simulink model "SF007A_SysFricLrng"  (R2013b)
settings: Solver=FixedStepDiscrete  SolverMode=SingleTasking  StartTime=0.0  StopTime=1  FixedStep=0.002  RelTol=1e-3
PostLoadFcn:
  | , if any(exist('dsrtsu_mdlpostloadfcn', 'file') == [2, 3, 6]), try dsrtsu_mdlpostloadfcn('Execute', bdroot); catch fprintf('Error in PostLoadFcn (dsrtsu_mdlpostloadfcn) for model "%s":\n %s\n', bdroot, lasterr); end, end,
values from neighbouring files (symbols this model uses):
  ARCHGLBPRM_100MILLISEC_SEC_F32 = DataDict.Constant    [SF007A_SysFricLrng_DataDict.m]
  ARCHGLBPRM_10MILLISEC_SEC_F32 = DataDict.Constant    [SF007A_SysFricLrng_DataDict.m]
  ARCHGLBPRM_180OVERPI_ULS_F32 = DataDict.Constant    [SF007A_SysFricLrng_DataDict.m]
  CONV100MICROSECTOSEC_ULS_F32 = DataDict.Constant    [SF007A_SysFricLrng_DataDict.m]
  FLTINJ_SYSFRICLRNG_SYSFRICOFFS = DataDict.Constant    [SF007A_SysFricLrng_DataDict.m]
  FricLrngData = DataDict.NVM    [SF007A_SysFricLrng_DataDict.m]
  HWPTNUM_CNT_U08 = DataDict.Constant    [SF007A_SysFricLrng_DataDict.m]
  HWPTNUMSUB1_CNT_U08 = DataDict.Constant    [SF007A_SysFricLrng_DataDict.m]
  HWVELDECDIR_ULS_U08 = DataDict.Constant    [SF007A_SysFricLrng_DataDict.m]
  HWVELINCDIR_ULS_U08 = DataDict.Constant    [SF007A_SysFricLrng_DataDict.m]
  IDXCALCNSCAGFAC_ULS_U08 = DataDict.Constant    [SF007A_SysFricLrng_DataDict.m]
  IDXSELN1_ULS_U08 = DataDict.Constant    [SF007A_SysFricLrng_DataDict.m]
  IDXSELN2_ULS_U08 = DataDict.Constant    [SF007A_SysFricLrng_DataDict.m]
  IDXSELN3_ULS_U08 = DataDict.Constant    [SF007A_SysFricLrng_DataDict.m]
  LRNGENASCAFAC_MILLISEC_U32 = DataDict.Constant    [SF007A_SysFricLrng_DataDict.m]
  SCAGFACQUARTER_CNT_F32 = DataDict.Constant    [SF007A_SysFricLrng_DataDict.m]
  SCAGFACTEN_CNT_U16 = DataDict.Constant    [SF007A_SysFricLrng_DataDict.m]
  SCAGFACVEHLATA_MTRPERSECSQD_F32 = DataDict.Constant    [SF007A_SysFricLrng_DataDict.m]
  SECIDXSELN_ULS_U08 = DataDict.Constant    [SF007A_SysFricLrng_DataDict.m]
  SysFricLrngBasLineEolFric = DataDict.Calibration    [SF007A_SysFricLrng_DataDict.m]
  SysFricLrngBasLineFric = DataDict.Calibration    [SF007A_SysFricLrng_DataDict.m]
  SysFricLrngBasLineHys = DataDict.Calibration    [SF007A_SysFricLrng_DataDict.m]
  SysFricLrngBasLineRngCntr = DataDict.Calibration    [SF007A_SysFricLrng_DataDict.m]
  SysFricLrngEolFricDifScagFac = DataDict.Calibration    [SF007A_SysFricLrng_DataDict.m]
  SysFricLrngFricChgWght = DataDict.Calibration    [SF007A_SysFricLrng_DataDict.m]
  SysFricLrngFricDiagcThd = DataDict.Calibration    [SF007A_SysFricLrng_DataDict.m]
  SysFricLrngFricDiagcTiThd = DataDict.Calibration    [SF007A_SysFricLrng_DataDict.m]
  SysFricLrngFricHysHwAgPt = DataDict.Calibration    [SF007A_SysFricLrng_DataDict.m]
  SysFricLrngGain = DataDict.Calibration    [SF007A_SysFricLrng_DataDict.m]
  SysFricLrngHwPosnAuthyThd = DataDict.Calibration    [SF007A_SysFricLrng_DataDict.m]
  SysFricLrngHwVelConstrLim = DataDict.Calibration    [SF007A_SysFricLrng_DataDict.m]
  SysFricLrngHwVelHiLim = DataDict.Calibration    [SF007A_SysFricLrng_DataDict.m]
  SysFricLrngHwVelLoLim = DataDict.Calibration    [SF007A_SysFricLrng_DataDict.m]
  SysFricLrngIgnCycFricChgLim = DataDict.Calibration    [SF007A_SysFricLrng_DataDict.m]
  SysFricLrngLatAHiLim = DataDict.Calibration    [SF007A_SysFricLrng_DataDict.m]
  SysFricLrngLatALoLim = DataDict.Calibration    [SF007A_SysFricLrng_DataDict.m]
  SysFricLrngMaskVehSpd = DataDict.Calibration    [SF007A_SysFricLrng_DataDict.m]
  SysFricLrngRngCntrThd = DataDict.Calibration    [SF007A_SysFricLrng_DataDict.m]
  SysFricLrngThd = DataDict.Calibration    [SF007A_SysFricLrng_DataDict.m]
  SysFricLrngTHiLim = DataDict.Calibration    [SF007A_SysFricLrng_DataDict.m]
  SysFricLrngTLoLim = DataDict.Calibration    [SF007A_SysFricLrng_DataDict.m]
  SysFricLrngVehSpd = DataDict.Calibration    [SF007A_SysFricLrng_DataDict.m]
  SYSFRICOFFSLIM_HWNWTMTR_F32 = DataDict.Constant    [SF007A_SysFricLrng_DataDict.m]
  VEHSPDPTNUM1_ULS_U08 = DataDict.Constant    [SF007A_SysFricLrng_DataDict.m]
  VEHSPDPTNUM2_ULS_U08 = DataDict.Constant    [SF007A_SysFricLrng_DataDict.m]
undefined symbols (not defined in the file or in its folder): NtcNr1, NtcSts1, SysFricLrngOperMod1
libraries: Fil x19, simulink x17, NxtrLim x10, NxtrAbslt x3, NxtrNvM x2, FixdToFloat x2, FloatToFixd x1, LnrIntrpn x1
(part 7 of 7)

== system SF007A_SysFricLrng/SysFricLrng/SysFricLrngPer1/RunningAndCalibrationModes/FricLearning/Calculate Average Friction/Raw Average Calculation/Update LPF/InitAvrgFricLpFil3 ==
  RawAvgFric : Inport
  Action Port : ActionPort  ActionType=case
  CopyRight2 : Subsystem  Description=|  mask(Copyright Information){none=on}
      | Copyright info block.                                               
      |                                                                     
      | Place copyright information at the top of every subsystem in design.
      mask prompts: none "No parameters"
      mask help: Place copyright information at the top of every subsystem in design.
      mask Display:
      | NxtrConf = 'Nexteer Confidential';
      | 
      | sys = bdroot; %handle for the current model ("system")
      | first = get_param(sys,'Created');
      | first = first(end-3:end);  %year is last four digits
      | 
      | last = get_param(sys,'LastModifiedDate');
      | if isempty(last)
      |     last = datestr(now,'yyyy');
      | else
      |     last = last(end-3:end);
      | end
      | 
      | if strcmp(first,last)
      |     fprintf('%s -- Copyright %s Nexteer',NxtrConf,first)
      | else
      |     fprintf('%s -- %s%s- %s Nexteer',NxtrConf,char(169),first,last)
      | end
  FilLpUpdOutp : Subsystem  mask(FilLpUpdOutp){StVar=AvrgFricLpFil3}
      mask prompts: StVar "State Variable:"
      mask help: Simulink implementation of the LPF_OpUpdate_f32_m macro.
      mask init: same as SF007A_SysFricLrng/SysFricLrng/SysFricLrngPer1/RunningAndCalibrationModes/Running Mode/If Action Subsystem/BlendingFricChg/FilLpUpdOutp
      settings: AttributesFormatString=StVar: %<StVar>
      mask Display:
      | port_label('input',1,'Inp')
      | port_label('output',1,'Outp')
      | text(0.2,0.8,'FilLpUpdOutp')
  FiltAvgFric : Outport
  wires:
  RawAvgFric/1 -> FilLpUpdOutp/1(Input)
  FilLpUpdOutp/1(Out1) -> FiltAvgFric/1

== system SF007A_SysFricLrng/SysFricLrng/SysFricLrngPer1/RunningAndCalibrationModes/FricLearning/Calculate Average Friction/Raw Average Calculation/Update LPF/InitAvrgFricLpFil4 ==
  RawAvgFric : Inport
  Action Port : ActionPort  ActionType=default
  CopyRight2 : Subsystem  Description=|  mask(Copyright Information){none=on}
      | Copyright info block.                                               
      |                                                                     
      | Place copyright information at the top of every subsystem in design.
      mask prompts: none "No parameters"
      mask help: Place copyright information at the top of every subsystem in design.
      mask Display:
      | NxtrConf = 'Nexteer Confidential';
      | 
      | sys = bdroot; %handle for the current model ("system")
      | first = get_param(sys,'Created');
      | first = first(end-3:end);  %year is last four digits
      | 
      | last = get_param(sys,'LastModifiedDate');
      | if isempty(last)
      |     last = datestr(now,'yyyy');
      | else
      |     last = last(end-3:end);
      | end
      | 
      | if strcmp(first,last)
      |     fprintf('%s -- Copyright %s Nexteer',NxtrConf,first)
      | else
      |     fprintf('%s -- %s%s- %s Nexteer',NxtrConf,char(169),first,last)
      | end
  FilLpUpdOutp : Subsystem  mask(FilLpUpdOutp){StVar=AvrgFricLpFil4}
      mask prompts: StVar "State Variable:"
      mask help: Simulink implementation of the LPF_OpUpdate_f32_m macro.
      mask init: same as SF007A_SysFricLrng/SysFricLrng/SysFricLrngPer1/RunningAndCalibrationModes/Running Mode/If Action Subsystem/BlendingFricChg/FilLpUpdOutp
      settings: AttributesFormatString=StVar: %<StVar>
      mask Display:
      | port_label('input',1,'Inp')
      | port_label('output',1,'Outp')
      | text(0.2,0.8,'FilLpUpdOutp')
  FiltAvgFric : Outport
  wires:
  RawAvgFric/1 -> FilLpUpdOutp/1(Input)
  FilLpUpdOutp/1(Out1) -> FiltAvgFric/1

== system SF007A_SysFricLrng/SysFricLrng/SysFricLrngPer1/RunningAndCalibrationModes/FricLearning/Range Counter Manager/Range Counter Control1/UpdateBaselineFric/CopyRight2 ==

== system SF007A_SysFricLrng/SysFricLrng/SysFricLrngPer1/RunningAndCalibrationModes/FricLearning/Range Counter Manager/Range Counter Threshold Calculation/Do Nothig/CopyRight2 ==

== system SF007A_SysFricLrng/SysFricLrng/SysFricLrngPer1/RunningAndCalibrationModes/FricLearning/Range Counter Manager/Range Counter Threshold Calculation/RangeCounterThreshExceeded/CopyRight2 ==

== system SF007A_SysFricLrng/SysFricLrng/SysFricLrngPer1/RunningAndCalibrationModes/LearningConstraint/ColTqconstraint/ColTqAryCalcn/12 Delay's Execution/CopyRight2 ==

== system SF007A_SysFricLrng/SysFricLrng/SysFricLrngPer1/RunningAndCalibrationModes/LearningConstraint/HwAngConstraint/Handwheel Angle Buffer/12 Delay's Execution/CopyRight2 ==

== system SF007A_SysFricLrng/SysFricLrng/SysFricLrngPer1/RunningAndCalibrationModes/LearningConstraint/HwVelConstraint/Handwheel Velocity Buffer/12 Delay's Execution/CopyRight2 ==

== system SF007A_SysFricLrng/SysFricLrng/SysFricLrngPer1/RunningAndCalibrationModes/LearningConstraint/HwVelConstraint/Range_Monotonicity Calculation/ AllGTZ/CopyRight2 ==

== system SF007A_SysFricLrng/SysFricLrng/SysFricLrngPer1/RunningAndCalibrationModes/LearningConstraint/HwVelConstraint/Range_Monotonicity Calculation/AllLTZ/CopyRight2 ==

== system SF007A_SysFricLrng/SysFricLrng/SysFricLrngPer1/RunningAndCalibrationModes/FricLearning/Calculate Average Friction/NTC FAIL/GetTiSpan100MicroSec32bit/No wrapping/CopyRight2 ==

== system SF007A_SysFricLrng/SysFricLrng/SysFricLrngPer1/RunningAndCalibrationModes/FricLearning/Calculate Average Friction/NTC FAIL/GetTiSpan100MicroSec32bit/Wrapping/CopyRight2 ==

== system SF007A_SysFricLrng/SysFricLrng/SysFricLrngPer1/RunningAndCalibrationModes/FricLearning/Calculate Average Friction/NTC FAIL/NTCFAIL/SetNtcSts/SetNtcSts ==
  note: Note:
      |
      | - "ISO Fault Debounce Design" Simulink block intent to use here for Simulation purpose only. Do not Code this block
  NtcNr : Inport
  NtcStInfo : Inport  Port=2
  NtcSts : Inport  Port=3
  DebStep : Inport  Port=4
  CopyRight2 : Subsystem  Description=|  mask(Copyright Information){none=on}
      | Copyright info block.                                               
      |                                                                     
      | Place copyright information at the top of every subsystem in design.
      mask prompts: none "No parameters"
      mask help: Place copyright information at the top of every subsystem in design.
      mask Display:
      | NxtrConf = 'Nexteer Confidential';
      | 
      | sys = bdroot; %handle for the current model ("system")
      | first = get_param(sys,'Created');
      | first = first(end-3:end);  %year is last four digits
      | 
      | last = get_param(sys,'LastModifiedDate');
      | if isempty(last)
      |     last = datestr(now,'yyyy');
      | else
      |     last = last(end-3:end);
      | end
      | 
      | if strcmp(first,last)
      |     fprintf('%s -- Copyright %s Nexteer',NxtrConf,first)
      | else
      |     fprintf('%s -- %s%s- %s Nexteer',NxtrConf,char(169),first,last)
      | end
  Data Store Write : DataStoreWrite  DataStoreName=Ntc0X0A2Qlfr
  Data Type Conversion4 : DataTypeConversion  OutDataTypeStr=Enum: SigQlfr1
  Ground : Ground
  ISO Fault Debounce Design : Stateflow chart  TreatAsAtomicUnit=on
      settings: AttributesFormatString=|
      | Simulation Purpose Only.
      | Do Not Code this block
      | Diagnostic Manager Owns this requirement
  Terminator : Terminator
  Terminator1 : Terminator
  wires:
  NtcStInfo/1 -> Terminator1/1
  NtcNr/1 -> Terminator/1
  DebStep/1 -> ISO Fault Debounce Design/2(DebStep)
  ISO Fault Debounce Design/1(Qualifier) -> Data Type Conversion4/1
  Ground/1 -> ISO Fault Debounce Design/3(SvcClr)
  Data Type Conversion4/1 -> Data Store Write/1
  NtcSts/1 -> ISO Fault Debounce Design/1(NtcSts)

== system SF007A_SysFricLrng/SysFricLrng/SysFricLrngPer1/RunningAndCalibrationModes/FricLearning/Calculate Average Friction/NTC PASS /SetNtcSts/SetNtcSts/CopyRight2 ==

== system SF007A_SysFricLrng/SysFricLrng/SysFricLrngPer1/RunningAndCalibrationModes/FricLearning/Calculate Average Friction/Raw Average Calculation/Update LPF/InitAvrgFricLpFil1/CopyRight2 ==

== system SF007A_SysFricLrng/SysFricLrng/SysFricLrngPer1/RunningAndCalibrationModes/FricLearning/Calculate Average Friction/Raw Average Calculation/Update LPF/InitAvrgFricLpFil1/FilLpUpdOutp ==
  Input : Inport
  Add : Sum
  Data Store Read : DataStoreRead  DataStoreName=AvrgFricLpFil1  DataStoreElements=AvrgFricLpFil1.FilSt#AvrgFricLpFil1.FilGain
  Data Store Write : DataStoreWrite  DataStoreName=AvrgFricLpFil1  DataStoreElements=AvrgFricLpFil1.FilSt
  Display1 : Display
  Display2 : Display
  Product : Product
  Subtract : Sum  Inputs=+-
  Out1 : Outport  OutDataTypeStr=single
  wires:
  Data Store Read/2 -> Display1/1, Product/2
  Add/1 -> Out1/1, Data Store Write/1
  Product/1 -> Add/2
  Subtract/1 -> Product/1
  Input/1 -> Subtract/1
  Data Store Read/1 -> Display2/1, Subtract/2, Add/1

== system SF007A_SysFricLrng/SysFricLrng/SysFricLrngPer1/RunningAndCalibrationModes/FricLearning/Calculate Average Friction/Raw Average Calculation/Update LPF/InitAvrgFricLpFil2/CopyRight2 ==

== system SF007A_SysFricLrng/SysFricLrng/SysFricLrngPer1/RunningAndCalibrationModes/FricLearning/Calculate Average Friction/Raw Average Calculation/Update LPF/InitAvrgFricLpFil2/FilLpUpdOutp ==
  Input : Inport
  Add : Sum
  Data Store Read : DataStoreRead  DataStoreName=AvrgFricLpFil2  DataStoreElements=AvrgFricLpFil2.FilSt#AvrgFricLpFil2.FilGain
  Data Store Write : DataStoreWrite  DataStoreName=AvrgFricLpFil2  DataStoreElements=AvrgFricLpFil2.FilSt
  Display1 : Display
  Display2 : Display
  Product : Product
  Subtract : Sum  Inputs=+-
  Out1 : Outport  OutDataTypeStr=single
  wires:
  Data Store Read/2 -> Display1/1, Product/2
  Add/1 -> Out1/1, Data Store Write/1
  Product/1 -> Add/2
  Subtract/1 -> Product/1
  Input/1 -> Subtract/1
  Data Store Read/1 -> Display2/1, Subtract/2, Add/1

== system SF007A_SysFricLrng/SysFricLrng/SysFricLrngPer1/RunningAndCalibrationModes/FricLearning/Calculate Average Friction/Raw Average Calculation/Update LPF/InitAvrgFricLpFil3/CopyRight2 ==

== system SF007A_SysFricLrng/SysFricLrng/SysFricLrngPer1/RunningAndCalibrationModes/FricLearning/Calculate Average Friction/Raw Average Calculation/Update LPF/InitAvrgFricLpFil3/FilLpUpdOutp ==
  Input : Inport
  Add : Sum
  Data Store Read : DataStoreRead  DataStoreName=AvrgFricLpFil3  DataStoreElements=AvrgFricLpFil3.FilSt#AvrgFricLpFil3.FilGain
  Data Store Write : DataStoreWrite  DataStoreName=AvrgFricLpFil3  DataStoreElements=AvrgFricLpFil3.FilSt
  Display1 : Display
  Display2 : Display
  Product : Product
  Subtract : Sum  Inputs=+-
  Out1 : Outport  OutDataTypeStr=single
  wires:
  Data Store Read/2 -> Display1/1, Product/2
  Add/1 -> Out1/1, Data Store Write/1
  Product/1 -> Add/2
  Subtract/1 -> Product/1
  Input/1 -> Subtract/1
  Data Store Read/1 -> Display2/1, Subtract/2, Add/1

== system SF007A_SysFricLrng/SysFricLrng/SysFricLrngPer1/RunningAndCalibrationModes/FricLearning/Calculate Average Friction/Raw Average Calculation/Update LPF/InitAvrgFricLpFil4/CopyRight2 ==

== system SF007A_SysFricLrng/SysFricLrng/SysFricLrngPer1/RunningAndCalibrationModes/FricLearning/Calculate Average Friction/Raw Average Calculation/Update LPF/InitAvrgFricLpFil4/FilLpUpdOutp ==
  Input : Inport
  Add : Sum
  Data Store Read : DataStoreRead  DataStoreName=AvrgFricLpFil4  DataStoreElements=AvrgFricLpFil4.FilSt#AvrgFricLpFil4.FilGain
  Data Store Write : DataStoreWrite  DataStoreName=AvrgFricLpFil4  DataStoreElements=AvrgFricLpFil4.FilSt
  Display1 : Display
  Display2 : Display
  Product : Product
  Subtract : Sum  Inputs=+-
  Out1 : Outport  OutDataTypeStr=single
  wires:
  Data Store Read/2 -> Display1/1, Product/2
  Add/1 -> Out1/1, Data Store Write/1
  Product/1 -> Add/2
  Subtract/1 -> Product/1
  Input/1 -> Subtract/1
  Data Store Read/1 -> Display2/1, Subtract/2, Add/1

== system SF007A_SysFricLrng/SysFricLrng/SysFricLrngPer1/RunningAndCalibrationModes/FricLearning/Calculate Average Friction/NTC FAIL/NTCFAIL/SetNtcSts/SetNtcSts/CopyRight2 ==

== stateflow chart SF007A_SysFricLrng/SysFricLrng/SysFricLrngPer1/RunningAndCalibrationModes/FricLearning/Calculate Average Friction/NTC FAIL/NTCFAIL/SetNtcSts/SetNtcSts/ISO Fault Debounce Design ==
  note: NTCSTS_PASSD           (0)
      | NTCSTS_FAILD             (1)
      | NTCSTS_PREPASSD   (2)
      | NTCSTS_PREFAILD     (3)
      |
      | SIGQLFR_NORES        (0)
      | SIGQLFR_PASSD         (1)
      | SIGQLFR_FAILD           (2)
  note: Pass Loop
  note: Fail Loop
  note: 
  (default) -> (junction 89)
  (junction 89) -> (junction 95) [order 1] : [NtcSts ==3]
  (junction 89) -> (junction 93) [order 2] : [NtcSts ==2]
  (junction 89) -> (junction 141) [order 3] : [NtcSts ==1]
      | { ErrAcc = 32767;
      | Qualifier =2;
      |  }
  (junction 89) -> (junction 141) [order 4] : [NtcSts ==0]
      | { ErrAcc = -32768;
      | Qualifier=1;
      | }
  (junction 95) -> (junction 103) [order 2]
  (junction 95) -> (junction 111) [order 1] : [ErrAcc <=0]
      | {ErrAcc = DebStep;}
  (junction 93) -> (junction 123) [order 2] : {
      | ErrAcc = ErrAcc - DebStep;
      | }
  (junction 93) -> (junction 123) [order 1] : [(ErrAcc - DebStep) <= -32768]
      | { ErrAcc = -32768;
      | Qualifier=1;
      | }
  (junction 103) -> (junction 111) [order 1] : [(ErrAcc + DebStep) <32767]
      | {ErrAcc = ErrAcc + DebStep;}
  (junction 103) -> (junction 111) [order 2] : {ErrAcc = 32767;
      | Qualifier =2;}
  (junction 123) -> (junction 141)
  (junction 111) -> (junction 141)
  (junction 141) -> (junction 159) [order 2] : {ErrAcc = 0;
      | Qualifier =0;
      | }
  (junction 141) -> (junction 159) [order 1] : [SvcClr ==0]
  data: NtcSts input Enum: NtcSts1; Qualifier output uint8; DebStep input uint16; ErrAcc local single; SvcClr input

== stateflow chart SF007A_SysFricLrng/SysFricLrng/SysFricLrngPer1/RunningAndCalibrationModes/FricLearning/Calculate Average Friction/NTC PASS /SetNtcSts/SetNtcSts/ISO Fault Debounce Design ==
  note: NTCSTS_PASSD           (0)
      | NTCSTS_FAILD             (1)
      | NTCSTS_PREPASSD   (2)
      | NTCSTS_PREFAILD     (3)
      |
      | SIGQLFR_NORES        (0)
      | SIGQLFR_PASSD         (1)
      | SIGQLFR_FAILD           (2)
  note: Pass Loop
  note: Fail Loop
  note: 
  (default) -> (junction 89)
  (junction 89) -> (junction 95) [order 1] : [NtcSts ==3]
  (junction 89) -> (junction 93) [order 2] : [NtcSts ==2]
  (junction 89) -> (junction 141) [order 3] : [NtcSts ==1]
      | { ErrAcc = 32767;
      | Qualifier =2;
      |  }
  (junction 89) -> (junction 141) [order 4] : [NtcSts ==0]
      | { ErrAcc = -32768;
      | Qualifier=1;
      | }
  (junction 95) -> (junction 103) [order 2]
  (junction 95) -> (junction 111) [order 1] : [ErrAcc <=0]
      | {ErrAcc = DebStep;}
  (junction 93) -> (junction 123) [order 2] : {
      | ErrAcc = ErrAcc - DebStep;
      | }
  (junction 93) -> (junction 123) [order 1] : [(ErrAcc - DebStep) <= -32768]
      | { ErrAcc = -32768;
      | Qualifier=1;
      | }
  (junction 103) -> (junction 111) [order 1] : [(ErrAcc + DebStep) <32767]
      | {ErrAcc = ErrAcc + DebStep;}
  (junction 103) -> (junction 111) [order 2] : {ErrAcc = 32767;
      | Qualifier =2;}
  (junction 123) -> (junction 141)
  (junction 111) -> (junction 141)
  (junction 141) -> (junction 159) [order 2] : {ErrAcc = 0;
      | Qualifier =0;
      | }
  (junction 141) -> (junction 159) [order 1] : [SvcClr ==0]
  data: NtcSts input Enum: NtcSts1; Qualifier output uint8; DebStep input uint16; ErrAcc local single; SvcClr input
